simulink model "inductor"  (R2020a)
settings: Solver=VariableStepAuto  StartTime=0.0  StopTime=tmax  FixedStep=1  MaxStep=dt  RelTol=1e-3
values from neighbouring files (symbols this model uses):
  Afe = (do-di)/2*h    (= 8.75e-05)    [run_inductor.m]    (also in run_inductor_sweep.m)
  am = 0.5    [run_inductor.m]    (also in run_inductor_sweep.m)
  B0 = -1    [run_inductor.m]    (also in run_inductor_sweep.m)
  cex = 0.3137    [run_inductor.m]    (also in run_inductor_sweep.m)
  d = 0.35e-3    (= 0.00035)    [run_inductor.m]    (also in run_inductor_sweep.m)
  delta = 0    [run_inductor.m]    (also in run_inductor_sweep.m)
  dens = 7650    [run_inductor.m]    (also in run_inductor_sweep.m)
  dt = deadtime/2    (= 5e-08)    [run_inductor.m]    (also in run_inductor_sweep.m = 0)
  f = 400    [run_inductor.m]    (also in run_inductor_sweep.m)
  lfe = (do+di)/2*pi    (= 0.359712358836)    [run_inductor.m]    (also in run_inductor_sweep.m)
  Lsig = 1.8735e-06    [run_inductor.m]    (also in run_inductor_sweep.m)
  N1 = 254    [run_inductor.m]    (also in run_inductor_sweep.m)
  nu0 = 1/mu0    (= 795774.715459)    [run_inductor.m]    (also in run_inductor_sweep.m)
  R = 0.56    [run_inductor.m]    (also in run_inductor_sweep.m)
  Rfe = N1^2*Afe/lfe/(sigma*d^2/12-C(1,2:end)*Cinv*C(2:end,1))    [run_inductor.m]    (also in run_inductor_sweep.m)
  sigma = 1/52e-8    (= 1923076.92308)    [run_inductor.m]    (also in run_inductor_sweep.m)
  Udc = 128.11    [run_inductor.m]    (also in run_inductor_sweep.m)
  uphase = 0    [run_inductor.m]    (also in run_inductor_sweep.m)
libraries: powerlib x12, powerlib_meascontrol x6
settings Model: Creator=rasilo  LastModifiedBy=wmartine
settings SolverCC: ZeroCrossAlgorithm=Adaptive
settings DataIOCC: ReturnWorkspaceOutputs=off
settings DebuggingCC: ArithmeticOperatorsInVariantConditions=warning
settings SFSimCC: SimUseLocalCustomCode=off  CustomCodeUndefinedFunction=UseInterfaceOnly
settings RTWCC: RTWUseLocalCustomCode=off
settings CodeAppCC: StateflowObjectComments=on
settings SimscapeCC: SimscapeNormalizeSystem=off

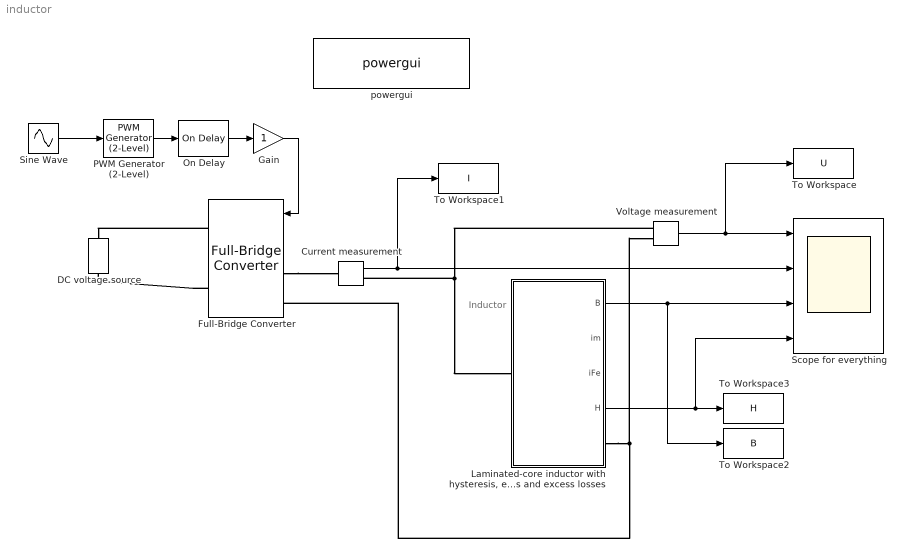
== system inductor ==
  note: Inductor
  Current measurement : powerlib/Measurements/Current Measurement  PhasorSimulation=off  OutputType=Complex  PSBequivalent=0
  DC voltage source : powerlib/Electrical Sources/DC Voltage Source  Amplitude=Udc  Measurements=None
  Full-Bridge Converter : powerlib/Power Electronics/Full-Bridge Converter  ModelType=Switching devices  Ron=55e-3  Rs=1e6  Cs=1e-6  Vforward=[0,0]  Ron_Diode=1e-3  Rs_Diode=1e6  Cs_Diode=inf  Vf_Diode=1e-3  Rs_CurrentSource=inf
      settings: SourceProductBaseCode=PS
  Gain : Gain
  "Laminated-core inductor with hysteresis, eddy currents and excess losses" : Subsystem
  On Delay : powerlib_meascontrol/Logic/On Delay  DelayType=On delay  delay=deadtime  ic=0  Ts=0
  PWM Generator (2-Level) : powerlib_meascontrol/Pulse & Signal Generators/PWM Generator (2-Level)  ModulatorType=Single-phase full-bridge (4 pulses)  ModulatorMode=Unsynchronized  Fc=fcar  Pc=0  nF=27  MinMax="[ -1  1 ]"  SamplingTechnique=Natural  ModulatingSignals=off  m=0.8  Freq=60  Phase=0  Ts=0  ShowCarrierOutport=off
  Scope for everything : Scope  NumInputPorts=4
  Sine Wave : Sin  Amplitude=am  Frequency=2*pi*f  Phase=uphase  SampleTime=0
  To Workspace : ToWorkspace  VariableName=U  SaveFormat=Structure With Time  SampleTime=-1
  To Workspace1 : ToWorkspace  VariableName=I  SaveFormat=Structure With Time  SampleTime=-1
  To Workspace2 : ToWorkspace  VariableName=B  SampleTime=-1
  To Workspace3 : ToWorkspace  VariableName=H  SampleTime=-1
  Voltage measurement : powerlib/Measurements/Voltage Measurement  PhasorSimulation=off  OutputType=Complex  PSBequivalent=0
  powergui : powerlib/powergui  Priority=1  SimulationMode=Discrete  SampleTime=dt  frequency=60  Iterations=50  frequencyindice=0  Pbase=100e6  ErrMax=1e-4  UnitsV=kV  UnitsW=MW  buscounter=0  FunctionMessages=off  echomessages=off  EnableUseOfTLC=off  CurrentSourceSwitches=off  DisableSnubberDevices=off  DisableRonSwitches=off  DisableVfSwitches=on  DisplayEquations=on  AutomaticDiscreteSolvers=off  SolverType=Backward Euler  Interpol=off  ExternalGateDelay=off  methode=off  Ts=0  x0status=blocks  SPID=off  SwTol=0  HookPort=off  NonlinearTolerance=1e-4  nMaxIteration=100  ContinueOnMaxIteration=off  RestoreLinks=warning  ResistiveCurrentMeasurement=off  Frange=[0:2:500]  Ylog=off  Xlog=on  ShowGrid=off  save=off  variable=ZData  structure=phase_a  ZoomFFT=off  StartTime=0.12  cycles=1  DisplayStyle=2  fundamental=50  FreqAxis=off  MaxFrequency=1000  frequencyindicesteady=1  RmsSteady=1  display=off
  wires:
  Current measurement/1 -> To Workspace1/1, Scope for everything/2
  Voltage measurement/1 -> To Workspace/1, Scope for everything/1
  "Laminated-core inductor with hysteresis, eddy currents and excess losses"/4(H) -> Scope for everything/4, To Workspace3/1
  "Laminated-core inductor with hysteresis, eddy currents and excess losses"/1(B) -> To Workspace2/1, Scope for everything/3
  PWM Generator (2-Level)/1 -> On Delay/1
  Gain/1 -> Full-Bridge Converter/1
  Sine Wave/1 -> PWM Generator (2-Level)/1
  On Delay/1 -> Gain/1
  connections:
  Voltage measurement/LConn1 -- "Laminated-core inductor with hysteresis, eddy currents and excess losses"/LConn1 -- Current measurement/RConn1
  Full-Bridge Converter/LConn1 -- Current measurement/LConn1
  "Laminated-core inductor with hysteresis, eddy currents and excess losses"/RConn1 -- Voltage measurement/LConn2 -- Full-Bridge Converter/LConn2
  Full-Bridge Converter/RConn1 -- DC voltage source/RConn1
  Full-Bridge Converter/RConn2 -- DC voltage source/LConn1

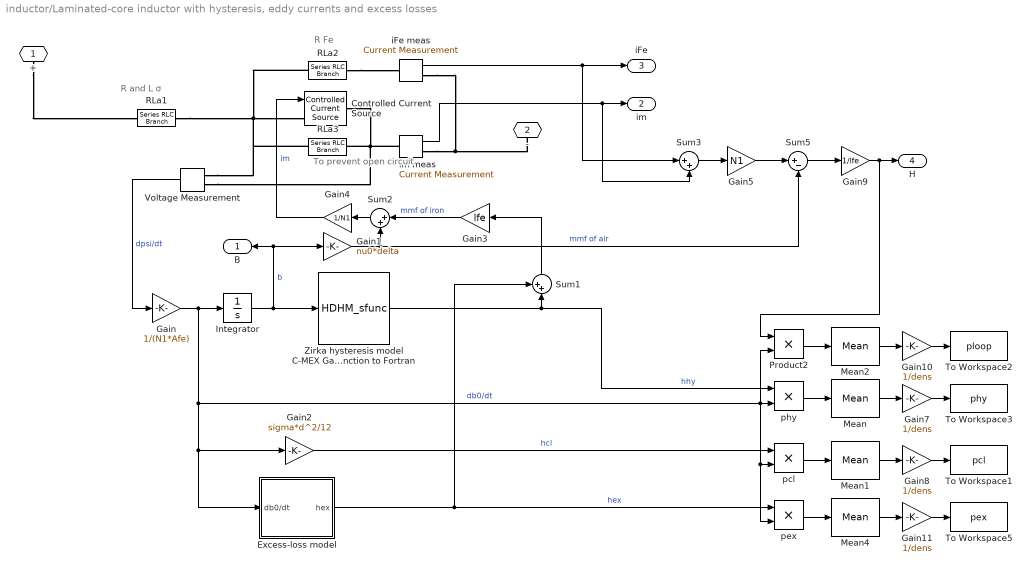
== system inductor/Laminated-core inductor with hysteresis, eddy currents and excess losses ==
  note: To prevent
      | open circuit
  note: R Fe
  note: R and L σ
  Controlled Current Source : powerlib/Electrical Sources/Controlled Current Source  Initialize=off  Source_Type=AC  Amplitude=0  Phase=0  Frequency=0  Measurements=None
  Excess-loss model : Subsystem
  Gain : Gain  Gain=1/(N1*Afe)
  Gain1 : Gain  Gain=nu0*delta
  Gain{7..8,10..11} (4 alike) : Gain  Gain=1/dens
  Gain2 : Gain  Gain=sigma*d^2/12
  Gain3 : Gain  Gain=lfe
  Gain4 : Gain  Gain=1/N1
  Gain5 : Gain  Gain=N1
  Gain9 : Gain  Gain=1/lfe
  Integrator : Integrator  InitialCondition=B0
  Mean{,1..2,4} (4 alike) : powerlib_meascontrol/Measurements/Mean  Freq=f  Vinit=0  Ts=0
  Product2 : Product
  RLa1 : powerlib/Elements/Series RLC Branch  LConnTagsString=__new0  RConnTagsString=__new0  BranchType=RL  Resistance=R  Inductance=Lsig  SetiL0=off  InitialCurrent=0  Capacitance=1e-6  Setx0=off  InitialVoltage=0  Measurements=None
  RLa2 : powerlib/Elements/Series RLC Branch  LConnTagsString=__new0  RConnTagsString=__new0  BranchType=R  Resistance=Rfe  Inductance=1e-3  SetiL0=off  InitialCurrent=0  Capacitance=1e-6  Setx0=off  InitialVoltage=0  Measurements=None
  RLa3 : powerlib/Elements/Series RLC Branch  LConnTagsString=__new0  RConnTagsString=__new0  BranchType=R  Resistance=100e3  Inductance=1e-3  SetiL0=off  InitialCurrent=0  Capacitance=1e-6  Setx0=off  InitialVoltage=0  Measurements=None
  Sum1 : Sum  Inputs=++|
  Sum2 : Sum  Inputs=|++
  Sum3 : Sum  Inputs=|++
  Sum5 : Sum  Inputs=|+-
  To Workspace1 : ToWorkspace  VariableName=pcl  SampleTime=-1
  To Workspace2 : ToWorkspace  VariableName=ploop  SampleTime=-1
  To Workspace3 : ToWorkspace  VariableName=phy  SampleTime=-1
  To Workspace5 : ToWorkspace  VariableName=pex  SampleTime=-1
  Voltage Measurement : powerlib/Measurements/Voltage Measurement  PhasorSimulation=off  OutputType=Complex  PSBequivalent=0
  Zirka hysteresis model C-MEX Gateway S-Function to Fortran : S-Function  FunctionName=HDHM_sfunc  Parameters=flag_hy  SFunctionDeploymentMode=off  EnableBusSupport=off
  iFe meas : powerlib/Measurements/Current Measurement  PhasorSimulation=off  OutputType=Complex  PSBequivalent=0
  im meas : powerlib/Measurements/Current Measurement  PhasorSimulation=off  OutputType=Complex  PSBequivalent=0
  pcl : Product
  pex : Product
  phy : Product
  + : PMIOPort  Side=Left
  - : PMIOPort  Port=2  Side=Right
  B : Outport
  im : Outport  Port=2
  iFe : Outport  Port=3
  H : Outport  Port=4
  wires:
  Integrator/1 -> B/1, Gain1/1, Zirka hysteresis model C-MEX Gateway S-Function to Fortran/1  "b"
  Voltage Measurement/1 -> Gain/1  "dpsi/dt"
  Gain2/1 -> pcl/1  "hcl"
  Gain4/1 -> Controlled Current Source/1  "im"
  Gain3/1 -> Sum2/1  "mmf of iron"
  Sum2/1 -> Gain4/1
  phy/1 -> Mean/1
  pcl/1 -> Mean1/1
  Gain1/1 -> Sum5/2, Sum2/2  "mmf of air"
  iFe meas/1 -> Sum3/1, iFe/1
  im meas/1 -> Sum3/2, im/1
  Sum3/1 -> Gain5/1
  Gain5/1 -> Sum5/1
  Sum5/1 -> Gain9/1
  Zirka hysteresis model C-MEX Gateway S-Function to Fortran/1 -> phy/1, Sum1/2  "hhy"
  Mean/1 -> Gain7/1
  Mean1/1 -> Gain8/1
  Gain7/1 -> To Workspace3/1
  Gain8/1 -> To Workspace1/1
  Product2/1 -> Mean2/1
  Gain9/1 -> Product2/1, H/1
  Mean2/1 -> Gain10/1
  Gain10/1 -> To Workspace2/1
  Gain/1 -> Integrator/1, Excess-loss model/1(db0/dt), Gain2/1, pex/2, pcl/2, Product2/2, phy/2  "db0/dt"
  Mean4/1 -> Gain11/1
  Gain11/1 -> To Workspace5/1
  pex/1 -> Mean4/1
  Sum1/1 -> Gain3/1
  Excess-loss model/1(hex) -> pex/1, Sum1/1  "hex"
  connections:
  im meas/RConn1 -- iFe meas/RConn1 -- -/RConn1
  RLa1/RConn1 -- RLa2/LConn1 -- Voltage Measurement/LConn1 -- RLa3/LConn1 -- Controlled Current Source/LConn1
  +/RConn1 -- RLa1/LConn1
  Voltage Measurement/LConn2 -- Controlled Current Source/RConn1 -- im meas/LConn1 -- RLa3/RConn1
  RLa2/RConn1 -- iFe meas/LConn1

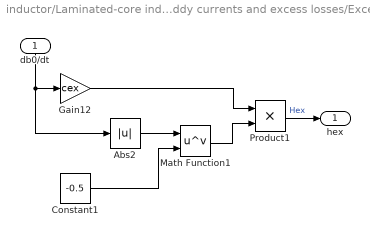
== system inductor/Laminated-core inductor with hysteresis, eddy currents and excess losses/Excess-loss model ==
  db0/dt : Inport
  Abs2 : Abs
  Constant1 : Constant  Value=-0.5
  Gain12 : Gain  Gain=cex
  Math Function1 : Math  Operator=pow  SignedPower=on  SaturateOnIntegerOverflow=on
  Product1 : Product
  hex : Outport
  wires:
  Constant1/1 -> Math Function1/2
  Abs2/1 -> Math Function1/1
  Math Function1/1 -> Product1/2
  Gain12/1 -> Product1/1
  Product1/1 -> hex/1  "Hex"
  db0/dt/1 -> Gain12/1, Abs2/1
